simulink model "TRAS_PID_Cross"  (Simulink 8.1)
settings: Solver=ode5  SolverMode=SingleTasking  StartTime=0.0  StopTime=90  FixedStep=0.01  RelTol=1e-3  AbsTol=1e-6
undefined symbols (not defined in the file): rtdac4pcibaseaddress
settings Model: Creator=jims  LastModifiedBy=inteco  SimulationMode=external  ExtModeTrigDuration=12000  ExtModeTrigLevel=0.400000
settings DataIOCC: ExternalInput=[]  InitialState=[]  LimitDataPoints=off  MaxDataPoints=5000  SaveOutput=off  SaveTime=off  SignalLoggingName=sigsOut
settings OptimizationCC: BooleanDataType=off  InitFltsAndDblsToZero=on
settings DebuggingCC: SaveWithParameterizedLinksMsg=none  MergeDetectMultiDrivingBlocksExec=error  SolverPrmCheckMsg=none  MultiTaskDSMMsg=warning  MultiTaskCondExecSysMsg=none  IntegerOverflowMsg=none  FcnCallInpInsideContextMsg=EnableAllAsWarning  StrictBusMsg=None
settings HardwareCC: TargetEndianess=LittleEndian  TargetHWDeviceType=MATLAB Host
settings RTWCC: SystemTargetFile=rtwin.tlc  TemplateMakefile=rtwin.tmf  Description=Real-Time Windows Target  ProcessScript=rtwin_make_rtw_hook  IncludeERTFirstTime=on
settings RTWinTargetCC: TargetFcnLib=ansi_tfl_tmw.mat  TargetLibSuffix=_rtwin.lib  TargetPreCompLibLocation=E:\apps_W32\MATLAB\R2013a\toolbox\rtw\targets\rtwin\lib\win32  CodeReplacementLibrary=ANSI_C  ModelReferenceCompliant=off  CompOptLevelCompliant=off  RTWinDir=E:/apps_W32/MATLAB/R2013a/toolbox/rtw/targets/rtwin  TargetArch=win32

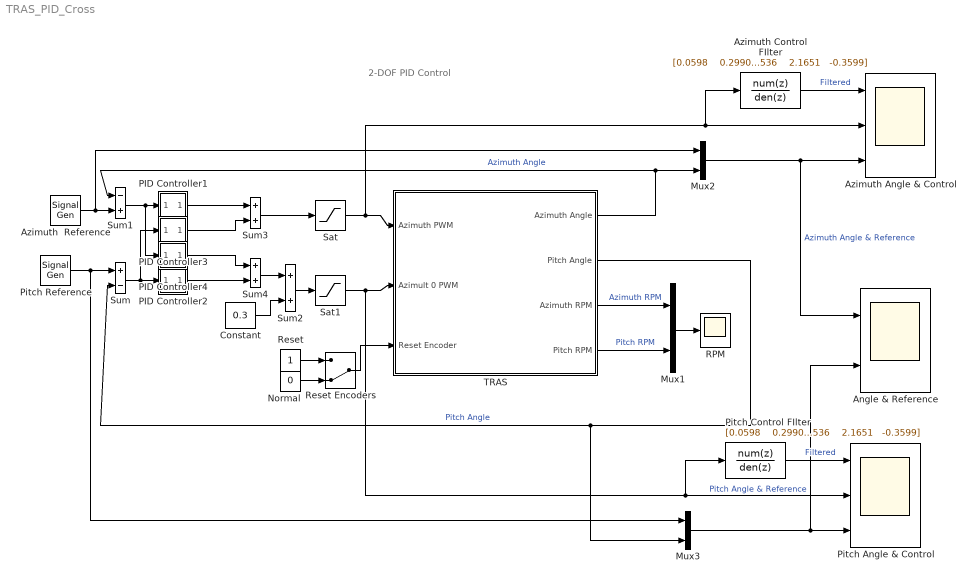
== system TRAS_PID_Cross ==
  note: 2-DOF PID Control
  Angle & Reference : Scope  NumInputPorts=2
      settings: TimeRange=90  YMin=-1~-0.5  YMax=1~0.4  SaveName=AngleReference_  MaxDataPoints=12000
  Azimuth Angle & Control : Scope  NumInputPorts=3
      settings: TimeRange=90  YMin=-0.4~-0.5~-1  YMax=-0.225~0.5~1  SaveName=AngleCtrl_  MaxDataPoints=12000
  Azimuth  Reference : SignalGenerator  WaveForm=square  Amplitude=.8  Frequency=.025
  Azimuth Control FIlter : DiscreteTransferFcn  Numerator="[0.0598    0.2990    0.5980    0.5980    0.2990    0.0598] * 1e-3"  Denominator="[1.0000   -3.9845    6.4349   -5.2536    2.1651   -0.3599]"  SampleTime=0.01
  Constant : Constant  Value=0.3
  Mux1 : Mux  Inputs=2
  Mux2 : Mux  Inputs=2
  Mux3 : Mux  Inputs=2
  Normal : Constant  Value=0
  PID Controller1 : Subsystem  mask(PID Controller){P=3.246, I=0.0367, D=2.152*2, S=1}
      mask prompts: P "Proportional:"; I "Integral:"; D "Derivative:"; S "Integral sat (0-1)"
      mask help:
      | Enter expressions for proportional, integral, and derivative terms.
      | P+I/s+Ds
      mask Help: This block implements a PID controller where parameters are entered for the Proportional, Integral and Derivative terms. Unmask this block to see how it works. The derivative term is implemented using a true derivative block.
      mask Display: disp('PID')
  PID Controller2 : Subsystem  mask(PID Controller){P=0.4978, I=0.4392, D=0.4464*2, S=1.43}
      mask prompts: P "Proportional:"; I "Integral:"; D "Derivative:"; S "Integral sat (0-1)"
      mask help:
      | Enter expressions for proportional, integral, and derivative terms.
      | P+I/s+Ds
      mask Help: This block implements a PID controller where parameters are entered for the Proportional, Integral and Derivative terms. Unmask this block to see how it works. The derivative term is implemented using a true derivative block.
      mask Display: disp('PID')
  PID Controller3 : Subsystem  mask(PID Controller){P=-0.9334, D=-0.7845}
      mask prompts: P "Proportional:"; D "Derivative:"
      mask help:
      | Enter expressions for proportional, integral, and derivative terms.
      | P+I/s+Ds
      mask Help: This block implements a PID controller where parameters are entered for the Proportional, Integral and Derivative terms. Unmask this block to see how it works. The derivative term is implemented using a true derivative block.
      mask Display: disp('PD')
  PID Controller4 : Subsystem  mask(PID Controller){P=-0.0363, D=-0.0223}
      mask prompts: P "Proportional:"; D "Derivative:"
      mask help:
      | Enter expressions for proportional, integral, and derivative terms.
      | P+I/s+Ds
      mask Help: This block implements a PID controller where parameters are entered for the Proportional, Integral and Derivative terms. Unmask this block to see how it works. The derivative term is implemented using a true derivative block.
      mask Display: disp('PD')
  Pitch Angle & Control : Scope  NumInputPorts=3
      settings: TimeRange=90  YMin=2.77556e-17~-0.1~-0.5  YMax=0.75~0.9~0.35  SaveName=AngleCtrl1_  MaxDataPoints=12000
  Pitch Reference : SignalGenerator  Amplitude=.3  Frequency=1/30
  Pitch Control FIlter : DiscreteTransferFcn  Numerator="[0.0598    0.2990    0.5980    0.5980    0.2990    0.0598] * 1e-3"  Denominator="[1.0000   -3.9845    6.4349   -5.2536    2.1651   -0.3599]"  SampleTime=0.01
  RPM : Scope
      settings: TimeRange=90  YMin=-6000  YMax=7000  SaveName=RPM_  MaxDataPoints=12000
  Reset : Constant
  Reset Encoders : ManualSwitch  CurrentSetting=0
  Sat : Saturate
  Sat1 : Saturate  UpperLimit=1  LowerLimit=-.2
  Sum : Sum  Inputs=+-  SaturateOnIntegerOverflow=on
  Sum1 : Sum  Inputs=-+  SaturateOnIntegerOverflow=on
  Sum2 : Sum  SaturateOnIntegerOverflow=on
  Sum3 : Sum  SaturateOnIntegerOverflow=on
  Sum4 : Sum  SaturateOnIntegerOverflow=on
  TRAS : Subsystem  mask{BaseAddress=rtdac4pcibaseaddress, T0=0.01}
      mask prompts: BaseAddress "Base Address:"; T0 "Sampling Period:"
      mask Display: image(imread('TRAS.JPG'))
  wires:
  Pitch Control FIlter/1 -> Pitch Angle & Control/1  "Filtered"
  Mux3/1 -> Pitch Angle & Control/3, Angle & Reference/2  "Pitch Angle & Reference"
  TRAS/2(Pitch Angle) -> Sum/2, Mux3/2  "Pitch Angle"
  Mux1/1 -> RPM/1
  PID Controller3/1(Out_1) -> Sum3/2
  PID Controller4/1(Out_1) -> Sum4/1
  PID Controller2/1(Out_1) -> Sum4/2
  Sum4/1 -> Sum2/1
  PID Controller1/1(Out_1) -> Sum3/1
  Sum3/1 -> Sat/1
  Constant/1 -> Sum2/2
  Sat/1 -> TRAS/1(Azimuth PWM), Azimuth Angle & Control/2, Azimuth Control FIlter/1
  Pitch Reference/1 -> Sum/1, Mux3/1
  Azimuth  Reference/1 -> Sum1/2, Mux2/1
  Sat1/1 -> TRAS/2(Azimult 0 PWM), Pitch Angle & Control/2, Pitch Control FIlter/1
  Sum2/1 -> Sat1/1
  Sum1/1 -> PID Controller4/1(In_1), PID Controller1/1(In_1)
  Sum/1 -> PID Controller2/1(In_1), PID Controller3/1(In_1)
  Azimuth Control FIlter/1 -> Azimuth Angle & Control/1  "Filtered"
  Mux2/1 -> Azimuth Angle & Control/3, Angle & Reference/1  "Azimuth Angle & Reference"
  Reset Encoders/1 -> TRAS/3(Reset Encoder)
  Reset/1 -> Reset Encoders/1
  Normal/1 -> Reset Encoders/2
  TRAS/4(Pitch RPM) -> Mux1/2  "Pitch RPM"
  TRAS/3(Azimuth RPM) -> Mux1/1  "Azimuth RPM"
  TRAS/1(Azimuth Angle) -> Sum1/1, Mux2/2  "Azimuth Angle"

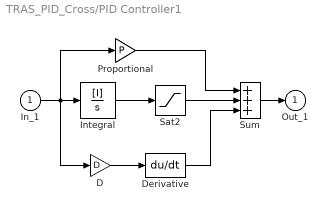
== system TRAS_PID_Cross/PID Controller1 ==
  In_1 : Inport
  D : Gain  Gain=D  SaturateOnIntegerOverflow=on  OutDataTypeStr=Inherit: Same as input  ParamDataTypeStr=Inherit: Same as input
  Derivative : Derivative
  Integral : TransferFcn  Numerator=[I]  Denominator=[1 0]
  Proportional : Gain  Gain=P  SaturateOnIntegerOverflow=on  OutDataTypeStr=Inherit: Same as input  ParamDataTypeStr=Inherit: Same as input
  Sat2 : Saturate  UpperLimit=S  LowerLimit=-S
  Sum : Sum  Inputs=+++  SaturateOnIntegerOverflow=on  InputSameDT=on  OutDataTypeStr=Inherit: Same as first input
  Out_1 : Outport  InitialOutput=0
  wires:
  Proportional/1 -> Sum/1
  Integral/1 -> Sat2/1
  Derivative/1 -> Sum/3
  In_1/1 -> Integral/1, Proportional/1, D/1
  Sum/1 -> Out_1/1
  D/1 -> Derivative/1
  Sat2/1 -> Sum/2

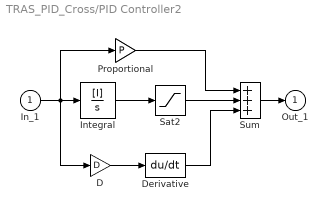
== system TRAS_PID_Cross/PID Controller2 ==
  In_1 : Inport
  D : Gain  Gain=D  SaturateOnIntegerOverflow=on  OutDataTypeStr=Inherit: Same as input  ParamDataTypeStr=Inherit: Same as input
  Derivative : Derivative
  Integral : TransferFcn  Numerator=[I]  Denominator=[1 0]
  Proportional : Gain  Gain=P  SaturateOnIntegerOverflow=on  OutDataTypeStr=Inherit: Same as input  ParamDataTypeStr=Inherit: Same as input
  Sat2 : Saturate  UpperLimit=S  LowerLimit=-S
  Sum : Sum  Inputs=+++  SaturateOnIntegerOverflow=on  InputSameDT=on  OutDataTypeStr=Inherit: Same as first input
  Out_1 : Outport  InitialOutput=0
  wires:
  Sat2/1 -> Sum/2
  D/1 -> Derivative/1
  Sum/1 -> Out_1/1
  In_1/1 -> D/1, Proportional/1, Integral/1
  Derivative/1 -> Sum/3
  Integral/1 -> Sat2/1
  Proportional/1 -> Sum/1

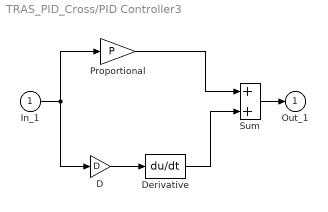
== system TRAS_PID_Cross/PID Controller3 ==
  In_1 : Inport
  D : Gain  Gain=D  SaturateOnIntegerOverflow=on  OutDataTypeStr=Inherit: Same as input  ParamDataTypeStr=Inherit: Same as input
  Derivative : Derivative
  Proportional : Gain  Gain=P  SaturateOnIntegerOverflow=on  OutDataTypeStr=Inherit: Same as input  ParamDataTypeStr=Inherit: Same as input
  Sum : Sum  SaturateOnIntegerOverflow=on  InputSameDT=on  OutDataTypeStr=Inherit: Same as first input
  Out_1 : Outport  InitialOutput=0
  wires:
  Derivative/1 -> Sum/2
  D/1 -> Derivative/1
  Sum/1 -> Out_1/1
  In_1/1 -> Proportional/1, D/1
  Proportional/1 -> Sum/1

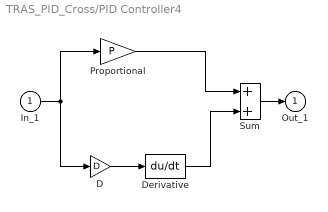
== system TRAS_PID_Cross/PID Controller4 ==
  In_1 : Inport
  D : Gain  Gain=D  SaturateOnIntegerOverflow=on  OutDataTypeStr=Inherit: Same as input  ParamDataTypeStr=Inherit: Same as input
  Derivative : Derivative
  Proportional : Gain  Gain=P  SaturateOnIntegerOverflow=on  OutDataTypeStr=Inherit: Same as input  ParamDataTypeStr=Inherit: Same as input
  Sum : Sum  SaturateOnIntegerOverflow=on  InputSameDT=on  OutDataTypeStr=Inherit: Same as first input
  Out_1 : Outport  InitialOutput=0
  wires:
  Proportional/1 -> Sum/1
  In_1/1 -> D/1, Proportional/1
  Sum/1 -> Out_1/1
  D/1 -> Derivative/1
  Derivative/1 -> Sum/2

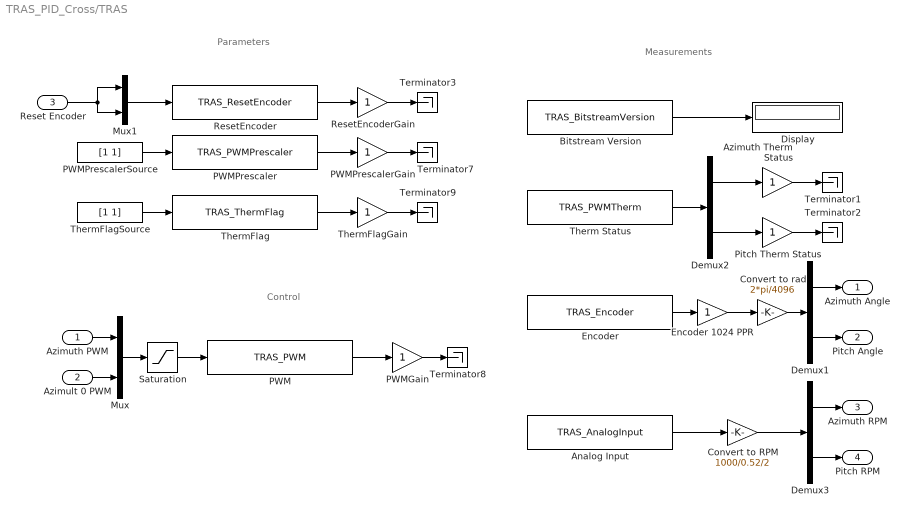
== system TRAS_PID_Cross/TRAS ==
  note: Parameters
  note: Control
  note: Measurements
  Azimuth PWM : Inport
  Azimult 0 PWM : Inport  Port=2
  Reset Encoder : Inport  Port=3
  Analog Input : S-Function  FunctionName=TRAS_AnalogInput  Parameters=BaseAddress, [1 0], [1 1], T0  EnableBusSupport=off
  Azimuth Therm Status : Gain  SaturateOnIntegerOverflow=on  OutDataTypeStr=Inherit: Same as input  ParamDataTypeStr=Inherit: Same as input
  Bitstream Version : S-Function  FunctionName=TRAS_BitstreamVersion  Parameters=BaseAddress, T0  EnableBusSupport=off
  Convert to RPM : Gain  Gain=1000/0.52/2  SaturateOnIntegerOverflow=on  OutDataTypeStr=Inherit: Same as input  ParamDataTypeStr=Inherit: Same as input
  Convert to rad : Gain  Gain=2*pi/4096  SaturateOnIntegerOverflow=on  OutDataTypeStr=Inherit: Same as input  ParamDataTypeStr=Inherit: Same as input
  Demux1 : Demux  Outputs=2
  Demux2 : Demux  Outputs=2
  Demux3 : Demux  Outputs=2
  Display : Display
  Encoder : S-Function  FunctionName=TRAS_Encoder  Parameters=BaseAddress, T0  EnableBusSupport=off
  Encoder 1024 PPR : Gain  SaturateOnIntegerOverflow=on  OutDataTypeStr=Inherit: Same as input  ParamDataTypeStr=Inherit: Same as input
  Mux : Mux  Inputs=2
  Mux1 : Mux  Inputs=2
  PWM : S-Function  FunctionName=TRAS_PWM  Parameters=BaseAddress, T0  EnableBusSupport=off
  PWMGain : Gain  SaturateOnIntegerOverflow=on  OutDataTypeStr=Inherit: Same as input  ParamDataTypeStr=Inherit: Same as input
  PWMPrescaler : S-Function  FunctionName=TRAS_PWMPrescaler  Parameters=BaseAddress, T0  EnableBusSupport=off
  PWMPrescalerGain : Gain  SaturateOnIntegerOverflow=on  OutDataTypeStr=Inherit: Same as input  ParamDataTypeStr=Inherit: Same as input
  PWMPrescalerSource : Constant  Value=[1 1]
  Pitch Therm Status : Gain  SaturateOnIntegerOverflow=on  OutDataTypeStr=Inherit: Same as input  ParamDataTypeStr=Inherit: Same as input
  ResetEncoder : S-Function  FunctionName=TRAS_ResetEncoder  Parameters=BaseAddress, T0  EnableBusSupport=off
  ResetEncoderGain : Gain  SaturateOnIntegerOverflow=on  OutDataTypeStr=Inherit: Same as input  ParamDataTypeStr=Inherit: Same as input
  Saturation : Saturate  UpperLimit=1  LowerLimit=-1
  Terminator{1..3,7..9} (6 alike) : Terminator
  Therm Status : S-Function  FunctionName=TRAS_PWMTherm  Parameters=BaseAddress, T0  EnableBusSupport=off
  "ThermFlag " : S-Function  FunctionName=TRAS_ThermFlag  Parameters=BaseAddress, T0  EnableBusSupport=off
  ThermFlagGain : Gain  SaturateOnIntegerOverflow=on  OutDataTypeStr=Inherit: Same as input  ParamDataTypeStr=Inherit: Same as input
  ThermFlagSource : Constant  Value=[1 1]
  Azimuth Angle : Outport  InitialOutput=0
  Pitch Angle : Outport  Port=2  InitialOutput=0
  Azimuth RPM : Outport  Port=3  InitialOutput=0
  Pitch RPM : Outport  Port=4  InitialOutput=0
  wires:
  Encoder 1024 PPR/1 -> Convert to rad/1
  Encoder/1 -> Encoder 1024 PPR/1
  Saturation/1 -> PWM/1
  Mux/1 -> Saturation/1
  PWM/1 -> PWMGain/1
  PWMGain/1 -> Terminator8/1
  ResetEncoder/1 -> ResetEncoderGain/1
  PWMPrescaler/1 -> PWMPrescalerGain/1
  Mux1/1 -> ResetEncoder/1
  PWMPrescalerSource/1 -> PWMPrescaler/1
  ResetEncoderGain/1 -> Terminator3/1
  PWMPrescalerGain/1 -> Terminator7/1
  Azimult 0 PWM/1 -> Mux/2
  Azimuth PWM/1 -> Mux/1
  Demux1/2 -> Pitch Angle/1
  Convert to rad/1 -> Demux1/1
  Demux1/1 -> Azimuth Angle/1
  Therm Status/1 -> Demux2/1
  Demux2/2 -> Pitch Therm Status/1
  Demux2/1 -> Azimuth Therm Status/1
  Azimuth Therm Status/1 -> Terminator1/1
  Pitch Therm Status/1 -> Terminator2/1
  Bitstream Version/1 -> Display/1
  Analog Input/1 -> Convert to RPM/1
  Demux3/2 -> Pitch RPM/1
  Demux3/1 -> Azimuth RPM/1
  Reset Encoder/1 -> Mux1/1, Mux1/2
  Convert to RPM/1 -> Demux3/1
  "ThermFlag "/1 -> ThermFlagGain/1
  ThermFlagSource/1 -> "ThermFlag "/1
  ThermFlagGain/1 -> Terminator9/1
